simulink model "HoppingRobotModel2"  (R2019b)
settings: Solver=VariableStepAuto  StartTime=0.0  StopTime=10.0  RelTol=1e-3
undefined symbols (not defined in the file): g, I1, I2, ini_theta1, ini_theta1_d, ini_theta2, ini_theta2_d, ini_w, ini_w_d, ini_x0, ini_x0_d, ini_y0, ini_y0_d, M1, M2, r1, r2
settings Model: Creator=fabia  LastModifiedBy=fabia

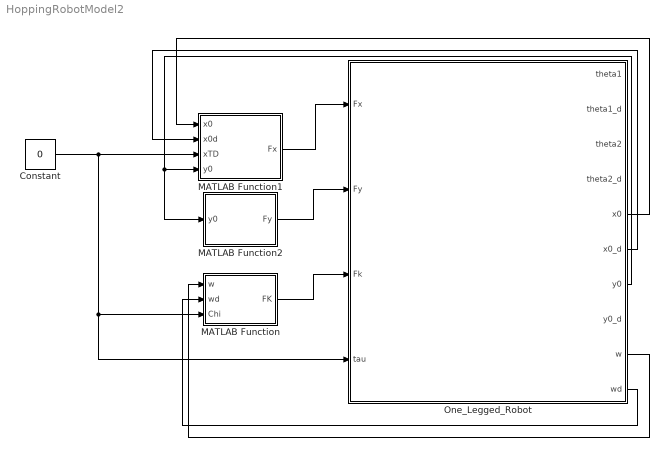
== system HoppingRobotModel2 ==
  Constant : Constant  Value=0
  MATLAB Function : MATLAB Function  TreatAsAtomicUnit=on
  MATLAB Function1 : MATLAB Function  TreatAsAtomicUnit=on
  MATLAB Function2 : MATLAB Function  TreatAsAtomicUnit=on
  One_Legged_Robot : Subsystem
  wires:
  One_Legged_Robot/5(x0) -> MATLAB Function1/1(x0)
  One_Legged_Robot/6(x0_d) -> MATLAB Function1/2(x0d)
  One_Legged_Robot/7(y0) -> MATLAB Function2/1(y0), MATLAB Function1/4(y0)
  One_Legged_Robot/9(w) -> MATLAB Function/1(w)
  One_Legged_Robot/10(wd) -> MATLAB Function/2(wd)
  Constant/1 -> One_Legged_Robot/4(tau), MATLAB Function/3(Chi), MATLAB Function1/3(xTD)
  MATLAB Function1/1(Fx) -> One_Legged_Robot/1(Fx)
  MATLAB Function2/1(Fy) -> One_Legged_Robot/2(Fy)
  MATLAB Function/1(FK) -> One_Legged_Robot/3(Fk)

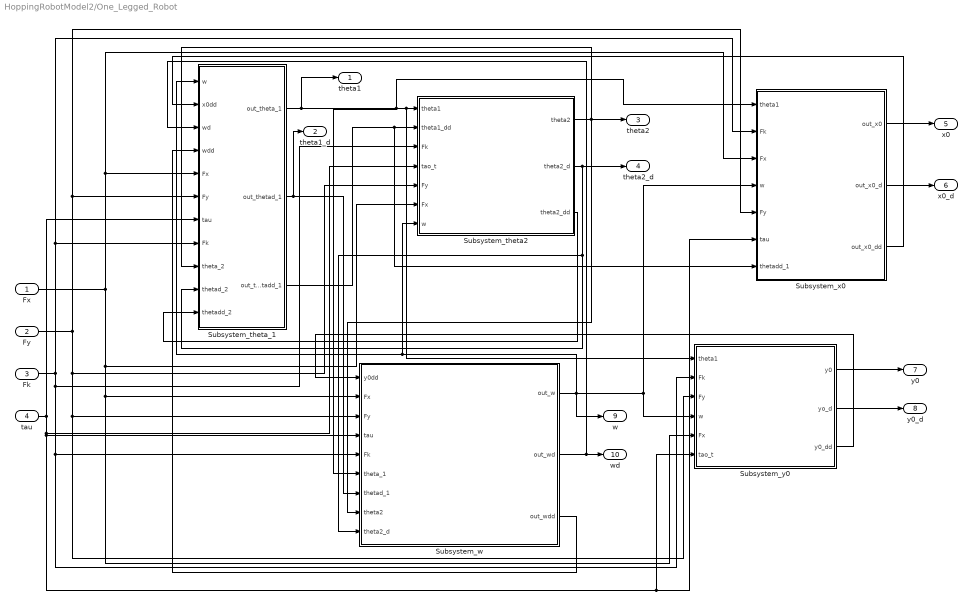
== system HoppingRobotModel2/One_Legged_Robot ==
  Fx : Inport
  Fy : Inport  Port=2
  Fk : Inport  Port=3
  tau : Inport  Port=4
  Subsystem_theta2 : Subsystem
  Subsystem_theta_1 : Subsystem
  Subsystem_w : Subsystem
  Subsystem_x0 : Subsystem
  Subsystem_y0 : Subsystem
  theta1 : Outport
  theta1_d : Outport  Port=2
  theta2 : Outport  Port=3
  theta2_d : Outport  Port=4
  x0 : Outport  Port=5
  x0_d : Outport  Port=6
  y0 : Outport  Port=7
  y0_d : Outport  Port=8
  w : Outport  Port=9
  wd : Outport  Port=10
  wires:
  Subsystem_theta_1/1(out_theta_1) -> theta1/1, Subsystem_y0/1(theta1), Subsystem_theta2/1(theta1), Subsystem_w/6(theta_1), Subsystem_x0/1(theta1)
  Subsystem_theta_1/3(out_thetadd_1) -> Subsystem_x0/7(thetadd_1), Subsystem_theta2/2(theta1_dd)
  Subsystem_theta_1/2(out_thetad_1) -> theta1_d/1, Subsystem_w/7(thetad_1)
  Subsystem_theta2/1(theta2) -> theta2/1, Subsystem_theta_1/9(theta_2), Subsystem_w/8(theta2)
  Subsystem_theta2/2(theta2_d) -> theta2_d/1, Subsystem_theta_1/10(thetad_2), Subsystem_w/9(theta2_d)
  Subsystem_theta2/3(theta2_dd) -> Subsystem_theta_1/11(thetadd_2)
  Subsystem_x0/3(out_x0_dd) -> Subsystem_theta_1/2(x0dd)
  Subsystem_w/1(out_w) -> w/1, Subsystem_x0/4(w), Subsystem_y0/4(w), Subsystem_theta2/7(w), Subsystem_theta_1/1(w)
  Subsystem_w/2(out_wd) -> wd/1, Subsystem_theta_1/3(wd)
  Subsystem_w/3(out_wdd) -> Subsystem_theta_1/4(wdd)
  Subsystem_y0/3(y0_dd) -> Subsystem_w/1(y0dd)
  Fx/1 -> Subsystem_x0/3("Fx "), Subsystem_theta_1/5(Fx), Subsystem_y0/5(Fx), Subsystem_w/2(Fx), Subsystem_theta2/6(Fx)
  Fy/1 -> Subsystem_x0/5("Fy "), Subsystem_theta_1/6(Fy), Subsystem_w/3(Fy), Subsystem_y0/3(Fy), Subsystem_theta2/5(Fy)
  Fk/1 -> Subsystem_w/5(Fk), Subsystem_y0/2(Fk), Subsystem_theta2/3(Fk), Subsystem_theta_1/8(Fk), Subsystem_x0/2(Fk)
  tau/1 -> Subsystem_theta_1/7(tau), Subsystem_y0/6(tao_t), Subsystem_x0/6(tau), Subsystem_w/4(tau), Subsystem_theta2/4(tao_t)
  Subsystem_x0/1("out_x0 ") -> x0/1
  Subsystem_x0/2(out_x0_d) -> x0_d/1
  Subsystem_y0/1(y0) -> y0/1
  Subsystem_y0/2(yo_d) -> y0_d/1

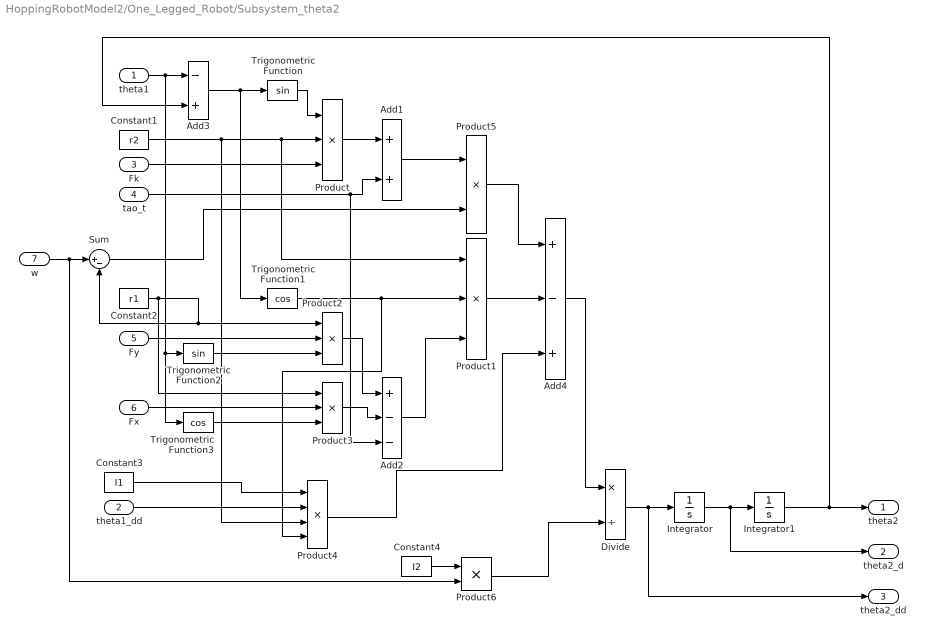
== system HoppingRobotModel2/One_Legged_Robot/Subsystem_theta2 ==
  theta1 : Inport
  theta1_dd : Inport  Port=2
  Fk : Inport  Port=3
  tao_t : Inport  Port=4
  Fy : Inport  Port=5
  Fx : Inport  Port=6
  w : Inport  Port=7
  Add1 : Sum
  Add2 : Sum  Inputs=+--
  Add3 : Sum  Inputs=-+
  Add4 : Sum  Inputs=+-+
  Constant1 : Constant  Value=r2
  Constant2 : Constant  Value=r1
  Constant3 : Constant  Value=I1
  Constant4 : Constant  Value=I2
  Divide : Product  Inputs=*/
  Integrator : Integrator  InitialCondition=ini_theta2_d
  Integrator1 : Integrator  InitialCondition=ini_theta2  LimitOutput=on  UpperSaturationLimit=pi/4  LowerSaturationLimit=-pi/4
  Product{,1..3} (4 alike) : Product  Inputs=3
  Product4 : Product  Inputs=4
  Product5 : Product
  Product6 : Product
  Sum : Sum  Inputs=|+-
  Trigonometric Function : Trigonometry
  Trigonometric Function1 : Trigonometry  Operator=cos
  Trigonometric Function2 : Trigonometry
  Trigonometric Function3 : Trigonometry  Operator=cos
  theta2 : Outport  VectorParamsAs1DForOutWhenUnconnected=off
  theta2_d : Outport  Port=2  VectorParamsAs1DForOutWhenUnconnected=off
  theta2_dd : Outport  Port=3  VectorParamsAs1DForOutWhenUnconnected=off
  wires:
  Fk/1 -> Product/3
  Product1/1 -> Add4/2
  Product2/1 -> Add2/1
  Product5/1 -> Add4/1
  Add4/1 -> Divide/1
  Add3/1 -> Trigonometric Function1/1, Trigonometric Function/1
  Trigonometric Function1/1 -> Product4/4, Product1/2
  Product/1 -> Add1/1
  Constant3/1 -> Product4/1
  Fx/1 -> Product3/2
  Add2/1 -> Product1/3
  Product3/1 -> Add2/2
  Constant1/1 -> Product4/3, Product1/1, Product/2
  Trigonometric Function3/1 -> Product3/3
  Constant2/1 -> Product3/1, Sum/2, Product2/1
  Trigonometric Function2/1 -> Product2/3
  Fy/1 -> Product2/2
  Integrator1/1 -> Add3/2, theta2/1
  Trigonometric Function/1 -> Product/1
  Add1/1 -> Product5/1
  tao_t/1 -> Add2/3, Add1/2
  theta1_dd/1 -> Product4/2
  theta1/1 -> Trigonometric Function3/1, Trigonometric Function2/1, Add3/1
  w/1 -> Product6/2, Sum/1
  Sum/1 -> Product5/2
  Product4/1 -> Add4/3
  Constant4/1 -> Product6/1
  Product6/1 -> Divide/2
  Divide/1 -> theta2_dd/1, Integrator/1
  Integrator/1 -> theta2_d/1, Integrator1/1

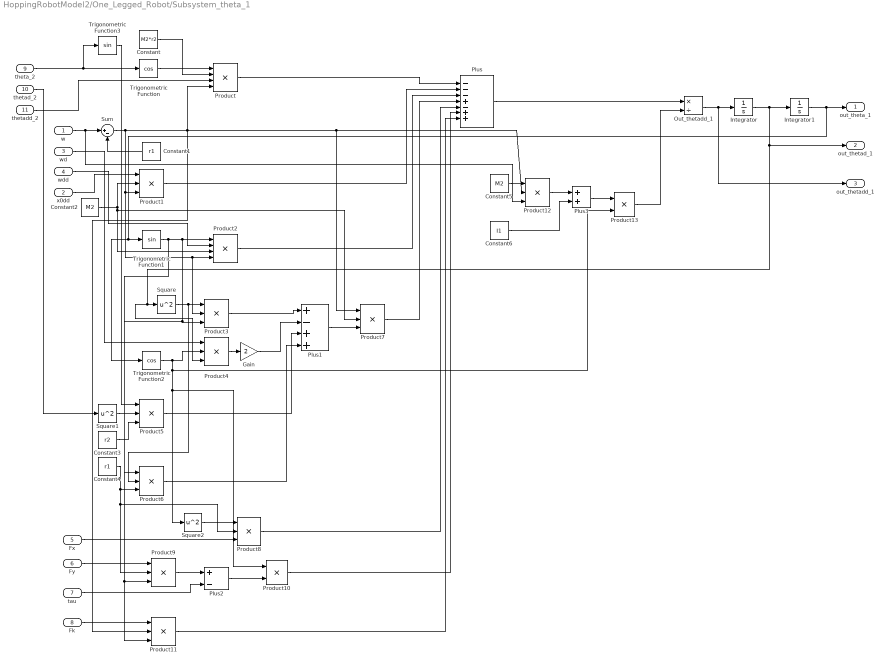
== system HoppingRobotModel2/One_Legged_Robot/Subsystem_theta_1 ==
  w : Inport
  x0dd : Inport  Port=2
  wd : Inport  Port=3
  wdd : Inport  Port=4
  Fx : Inport  Port=5
  Fy : Inport  Port=6
  tau : Inport  Port=7
  Fk : Inport  Port=8
  theta_2 : Inport  Port=9
  thetad_2 : Inport  Port=10
  thetadd_2 : Inport  Port=11
  Constant : Constant  Value=M2*r2
  Constant1 : Constant  Value=r1
  Constant2 : Constant  Value=M2
  Constant3 : Constant  Value=r2
  Constant4 : Constant  Value=r1
  Constant5 : Constant  Value=M2
  Constant6 : Constant  Value=I1
  Gain : Gain  Gain=2
  Integrator : Integrator  InitialCondition=ini_theta1_d
  Integrator1 : Integrator  InitialCondition=ini_theta1  LimitOutput=on  UpperSaturationLimit=pi/4  LowerSaturationLimit=-pi/4
  Out_thetadd_1 : Product  Inputs=*/
  Plus : Sum  Inputs=---+-++
  Plus1 : Sum  Inputs=+-++
  Plus2 : Sum  Inputs=+-
  Plus3 : Sum
  Product : Product  Inputs=4
  Product{1,3..9,11..12} (10 alike) : Product  Inputs=3
  Product10 : Product
  Product13 : Product
  Product2 : Product  Inputs=4
  Square : Math  Operator=square  SignedPower=off  SaturateOnIntegerOverflow=on
  Square1 : Math  Operator=square  SignedPower=off  SaturateOnIntegerOverflow=on
  Square2 : Math  Operator=square  SignedPower=off  SaturateOnIntegerOverflow=on
  Sum : Sum  Inputs=|+-
  Trigonometric Function : Trigonometry  Operator=cos
  Trigonometric Function1 : Trigonometry
  Trigonometric Function2 : Trigonometry  Operator=cos
  Trigonometric Function3 : Trigonometry
  out_theta_1 : Outport
  out_thetad_1 : Outport  Port=2
  out_thetadd_1 : Outport  Port=3
  wires:
  Trigonometric Function/1 -> Product/1
  Constant/1 -> Product/2
  Out_thetadd_1/1 -> out_thetadd_1/1, Integrator/1
  w/1 -> Product12/3, Sum/1
  Sum/1 -> Product2/4, Product3/2, Product1/3, Product11/2, Product12/2, Product7/1, Product/4
  x0dd/1 -> Product1/1
  Constant2/1 -> Product7/2, Product2/3, Product1/2
  Product/1 -> Plus/1
  Product1/1 -> Plus/2
  Trigonometric Function1/1 -> Product9/3, Product11/3, Product6/1, Product3/3, Product2/1
  Integrator1/1 -> Trigonometric Function2/1, Trigonometric Function1/1, out_theta_1/1
  wdd/1 -> Product2/2
  Product2/1 -> Plus/3
  Constant1/1 -> Sum/2
  Square/1 -> Product6/2, Product3/1
  Integrator/1 -> out_thetad_1/1, Product4/3, Square/1, Integrator1/1
  Product3/1 -> Plus1/1
  wd/1 -> Product4/1
  Trigonometric Function2/1 -> Product4/2, Product13/2, Product10/1, Square2/1
  Product4/1 -> Gain/1
  Gain/1 -> Plus1/2
  Trigonometric Function3/1 -> Product5/1
  Square1/1 -> Product5/2
  Constant3/1 -> Product5/3
  Product5/1 -> Plus1/3
  Constant4/1 -> Product9/2, Product8/2, Product6/3
  Product6/1 -> Plus1/4
  Plus1/1 -> Product7/3
  Product7/1 -> Plus/4
  Square2/1 -> Product8/1
  Fx/1 -> Product8/3
  Product8/1 -> Plus/5
  Fy/1 -> Product9/1
  Product9/1 -> Plus2/1
  tau/1 -> Plus2/2
  Plus2/1 -> Product10/2
  Product10/1 -> Plus/6
  Fk/1 -> Product11/1
  Product11/1 -> Plus/7
  Plus/1 -> Out_thetadd_1/1
  Constant5/1 -> Product12/1
  Product12/1 -> Plus3/1
  Constant6/1 -> Plus3/2
  Plus3/1 -> Product13/1
  Product13/1 -> Out_thetadd_1/2
  thetadd_2/1 -> Product/3
  theta_2/1 -> Trigonometric Function3/1, Trigonometric Function/1
  thetad_2/1 -> Square1/1

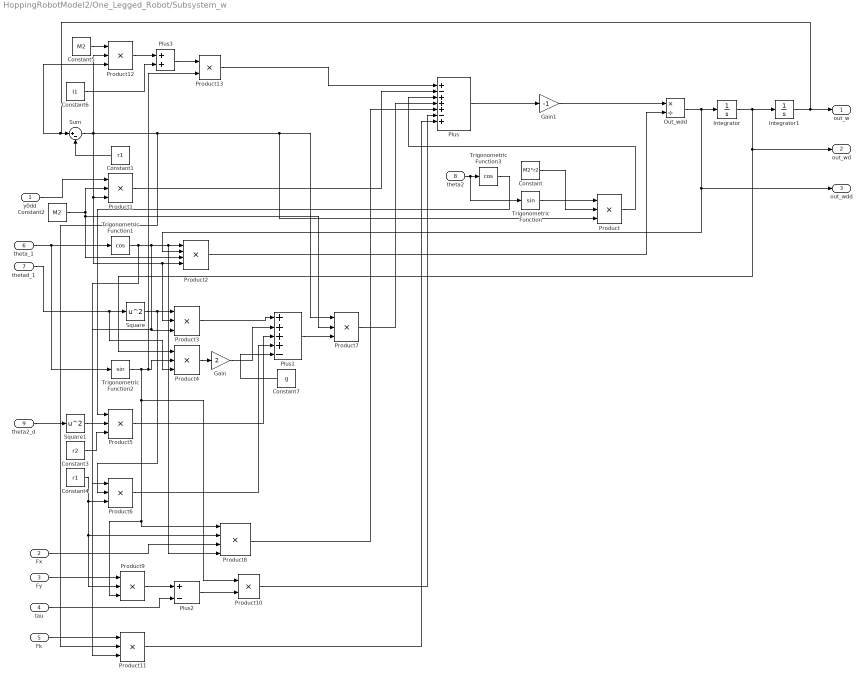
== system HoppingRobotModel2/One_Legged_Robot/Subsystem_w ==
  y0dd : Inport
  Fx : Inport  Port=2
  Fy : Inport  Port=3
  tau : Inport  Port=4
  Fk : Inport  Port=5
  theta_1 : Inport  Port=6
  thetad_1 : Inport  Port=7
  theta2 : Inport  Port=8
  theta2_d : Inport  Port=9
  Constant : Constant  Value=M2*r2
  Constant1 : Constant  Value=r1
  Constant2 : Constant  Value=M2
  Constant3 : Constant  Value=r2
  Constant4 : Constant  Value=r1
  Constant5 : Constant  Value=M2
  Constant6 : Constant  Value=I1
  Constant7 : Constant  Value=g
  Gain : Gain  Gain=2
  Gain1 : Gain  Gain=-1
  Integrator : Integrator  InitialCondition=ini_w_d
  Integrator1 : Integrator  InitialCondition=ini_w  UpperSaturationLimit=pi/4  LowerSaturationLimit=-pi/4
  Out_wdd : Product  Inputs=*/
  Plus : Sum  Inputs=+-+++-+
  Plus1 : Sum  Inputs=++++-
  Plus2 : Sum  Inputs=+-
  Plus3 : Sum
  Product{,1,3..7,9,11..12} (10 alike) : Product  Inputs=3
  Product10 : Product
  Product13 : Product
  Product2 : Product  Inputs=4
  Product8 : Product  Inputs=4
  Square : Math  Operator=square  SignedPower=off  SaturateOnIntegerOverflow=on
  Square1 : Math  Operator=square  SignedPower=off  SaturateOnIntegerOverflow=on
  Sum : Sum  Inputs=|+-
  Trigonometric Function : Trigonometry
  Trigonometric Function1 : Trigonometry  Operator=cos
  Trigonometric Function2 : Trigonometry
  Trigonometric Function3 : Trigonometry  Operator=cos
  out_w : Outport
  out_wd : Outport  Port=2
  out_wdd : Outport  Port=3
  wires:
  Integrator1/1 -> Product12/3, Sum/1, out_w/1
  Sum/1 -> Product12/2, Product2/4, Product3/2, Product1/3, Product11/2, Product/3, Product7/1
  y0dd/1 -> Product1/1
  Constant2/1 -> Product7/2, Product2/3, Product1/2
  Product1/1 -> Plus/2
  Trigonometric Function1/1 -> Product2/1, Product8/4, Product6/1, Product3/3, Product11/3
  Out_wdd/1 -> out_wdd/1, Product2/2, Integrator/1
  Constant1/1 -> Sum/2
  Square/1 -> Product6/2, Product3/1
  Product3/1 -> Plus1/1
  Integrator/1 -> Product4/1, out_wd/1, Integrator1/1
  Product4/1 -> Gain/1
  Gain/1 -> Plus1/2
  Square1/1 -> Product5/2
  Constant3/1 -> Product5/3
  Product5/1 -> Plus1/3
  Constant4/1 -> Product9/2, Product8/2, Product6/3
  Product6/1 -> Plus1/4
  Plus1/1 -> Product7/3
  Product7/1 -> Plus/4
  Trigonometric Function2/1 -> Product13/2, Product4/2, Product9/3, Product8/1, Product10/1
  Fx/1 -> Product8/3
  Product8/1 -> Plus/5
  Fy/1 -> Product9/1
  Product9/1 -> Plus2/1
  tau/1 -> Plus2/2
  Plus2/1 -> Product10/2
  Product10/1 -> Plus/6
  Fk/1 -> Product11/1
  Product11/1 -> Plus/7
  Constant5/1 -> Product12/1
  Product12/1 -> Plus3/1
  Plus3/1 -> Product13/1
  Constant/1 -> Product/2
  Constant6/1 -> Plus3/2
  theta_1/1 -> Trigonometric Function2/1, Trigonometric Function1/1
  thetad_1/1 -> Product4/3, Square/1
  Product13/1 -> Plus/1
  Trigonometric Function/1 -> Product/1
  Trigonometric Function3/1 -> Product5/1
  Constant7/1 -> Plus1/5
  Plus/1 -> Gain1/1
  Gain1/1 -> Out_wdd/1
  theta2/1 -> Trigonometric Function/1, Trigonometric Function3/1
  theta2_d/1 -> Square1/1
  Product/1 -> Plus/3
  Product2/1 -> Out_wdd/2

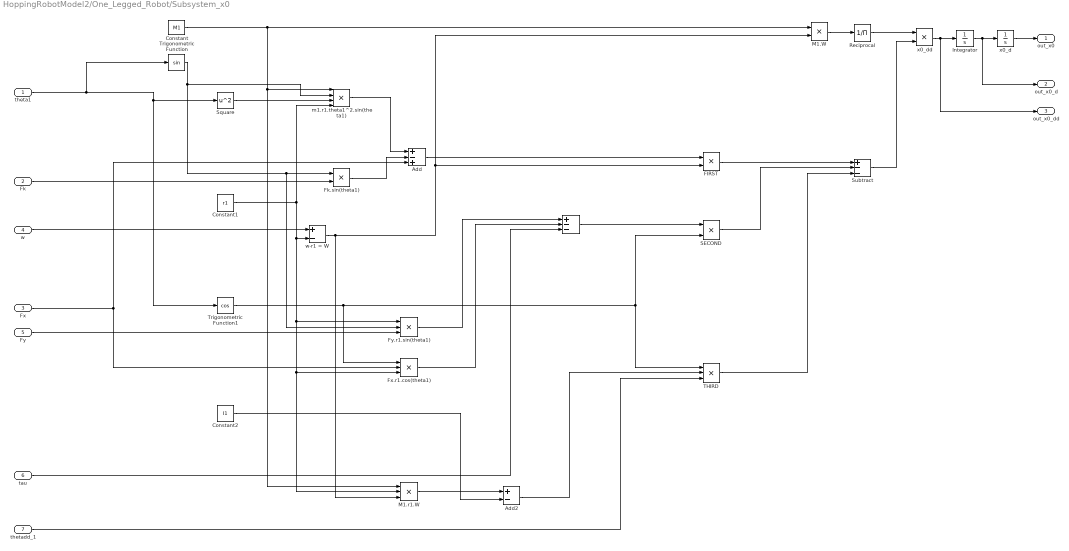
== system HoppingRobotModel2/One_Legged_Robot/Subsystem_x0 ==
  theta1 : Inport
  Fk : Inport  Port=2
  "Fx " : Inport  Port=3
  w : Inport  Port=4
  "Fy " : Inport  Port=5
  tau : Inport  Port=6
  thetadd_1 : Inport  Port=7
  " SECOND" : Product
  " " : Sum  Inputs=+--
  Add : Sum  Inputs=+-+
  Add2 : Sum  Inputs=+-
  Constant : Constant  Value=M1
  Constant1 : Constant  Value=r1
  Constant2 : Constant  Value=I1
  FIRST : Product
  Fk.sin(theta1) : Product
  Fx.r1.cos(theta1) : Product  Inputs=3
  Fy.r1.sin(theta1) : Product  Inputs=3
  Integrator : Integrator  InitialCondition=ini_x0_d
  M1.W : Product
  M1.r1.W : Product  Inputs=3
  Reciprocal : Product  Inputs=/
  Square : Math  Operator=square  SignedPower=off  SaturateOnIntegerOverflow=on
  Subtract : Sum  Inputs=+--
  "THIRD " : Product  Inputs=3
  Trigonometric Function : Trigonometry
  Trigonometric Function1 : Trigonometry  Operator=cos
  m1.r1.theta1^2.sin(theta1) : Product  Inputs=4
  w-r1 = W : Sum  Inputs=+-
  x0_d : Integrator  InitialCondition=ini_x0
  "x0_dd " : Product
  "out_x0 " : Outport
  out_x0_d : Outport  Port=2
  out_x0_dd : Outport  Port=3
  wires:
  Add/1 -> FIRST/1
  Constant1/1 -> m1.r1.theta1^2.sin(theta1)/4, M1.r1.W/2, Fx.r1.cos(theta1)/3, Fy.r1.sin(theta1)/1, w-r1 = W/2
  w/1 -> w-r1 = W/1
  Reciprocal/1 -> "x0_dd "/1
  thetadd_1/1 -> "THIRD "/3
  Trigonometric Function1/1 -> "THIRD "/1, " SECOND"/2, Fx.r1.cos(theta1)/1
  m1.r1.theta1^2.sin(theta1)/1 -> Add/1
  tau/1 -> " "/3
  M1.r1.W/1 -> Add2/1
  Square/1 -> m1.r1.theta1^2.sin(theta1)/3
  Trigonometric Function/1 -> Fy.r1.sin(theta1)/2, Fk.sin(theta1)/1, m1.r1.theta1^2.sin(theta1)/2
  Constant/1 -> m1.r1.theta1^2.sin(theta1)/1, M1.r1.W/1, M1.W/1
  Constant2/1 -> Add2/2
  FIRST/1 -> Subtract/1
  theta1/1 -> Trigonometric Function1/1, Square/1, Trigonometric Function/1
  "x0_dd "/1 -> out_x0_dd/1, Integrator/1
  "Fx "/1 -> Fx.r1.cos(theta1)/2, Add/3
  Fx.r1.cos(theta1)/1 -> " "/2
  x0_d/1 -> "out_x0 "/1
  w-r1 = W/1 -> FIRST/2, M1.W/2, M1.r1.W/3
  Add2/1 -> "THIRD "/2
  Integrator/1 -> out_x0_d/1, x0_d/1
  Fy.r1.sin(theta1)/1 -> " "/1
  "Fy "/1 -> Fy.r1.sin(theta1)/3
  M1.W/1 -> Reciprocal/1
  "THIRD "/1 -> Subtract/3
  " SECOND"/1 -> Subtract/2
  Fk/1 -> Fk.sin(theta1)/2
  Fk.sin(theta1)/1 -> Add/2
  " "/1 -> " SECOND"/1
  Subtract/1 -> "x0_dd "/2

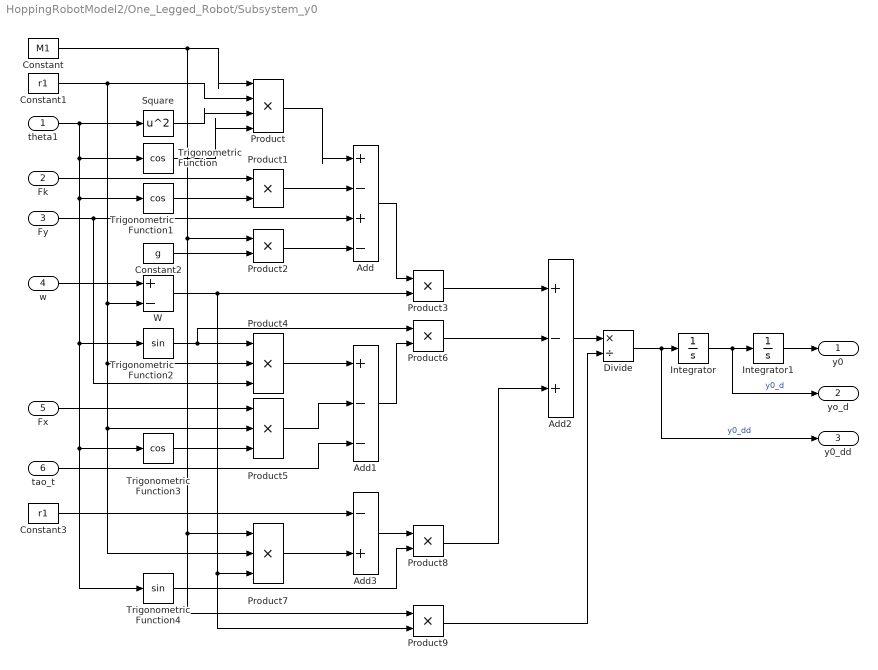
== system HoppingRobotModel2/One_Legged_Robot/Subsystem_y0 ==
  theta1 : Inport
  Fk : Inport  Port=2
  Fy : Inport  Port=3
  w : Inport  Port=4
  Fx : Inport  Port=5
  tao_t : Inport  Port=6
  Add : Sum  Inputs=+-+-
  Add1 : Sum  Inputs=+--
  Add2 : Sum  Inputs=+-+
  Add3 : Sum  Inputs=-+
  Constant : Constant  Value=M1
  Constant1 : Constant  Value=r1
  Constant2 : Constant  Value=g
  Constant3 : Constant  Value=r1
  Divide : Product  Inputs=*/
  Integrator : Integrator  InitialCondition=ini_y0_d
  Integrator1 : Integrator  InitialCondition=ini_y0
  Product : Product  Inputs=4
  Product{1..3,6,8..9} (6 alike) : Product
  Product4 : Product  Inputs=3
  Product5 : Product  Inputs=3
  Product7 : Product  Inputs=3
  Square : Math  Operator=square  SaturateOnIntegerOverflow=on
  Trigonometric Function : Trigonometry  Operator=cos
  Trigonometric Function1 : Trigonometry  Operator=cos
  Trigonometric Function2 : Trigonometry
  Trigonometric Function3 : Trigonometry  Operator=cos
  Trigonometric Function4 : Trigonometry
  W : Sum  Inputs=+-
  y0 : Outport  VectorParamsAs1DForOutWhenUnconnected=off
  yo_d : Outport  Port=2  VectorParamsAs1DForOutWhenUnconnected=off
  y0_dd : Outport  Port=3  VectorParamsAs1DForOutWhenUnconnected=off
  wires:
  Integrator/1 -> yo_d/1, Integrator1/1  "y0_d"
  Add2/1 -> Divide/1
  Square/1 -> Product/3
  Integrator1/1 -> y0/1
  Divide/1 -> y0_dd/1, Integrator/1  "y0_dd"
  Product8/1 -> Add2/3
  Product6/1 -> Add2/2
  Add3/1 -> Product8/1
  Trigonometric Function4/1 -> Product8/2
  Product7/1 -> Add3/2
  Product9/1 -> Divide/2
  Add1/1 -> Product6/2
  W/1 -> Product7/3, Product9/2, Product3/2
  Constant2/1 -> Product2/2
  Trigonometric Function1/1 -> Product1/2
  Product/1 -> Add/1
  Fy/1 -> Product4/3, Add/3
  w/1 -> W/1
  Add/1 -> Product3/1
  Fk/1 -> Product1/1
  Product4/1 -> Add1/1
  Fx/1 -> Product5/1
  Product1/1 -> Add/2
  Constant/1 -> Product9/1, Product7/1, Product2/1, Product/1
  Trigonometric Function/1 -> Product/4
  Trigonometric Function3/1 -> Product5/3
  Constant1/1 -> Product7/2, Product5/2, Product4/2, W/2, Product/2
  Product2/1 -> Add/4
  tao_t/1 -> Add1/3
  Trigonometric Function2/1 -> Product6/1, Product4/1
  Product5/1 -> Add1/2
  Constant3/1 -> Add3/1
  theta1/1 -> Trigonometric Function4/1, Trigonometric Function3/1, Trigonometric Function2/1, Trigonometric Function1/1, Trigonometric Function/1, Square/1
  Product3/1 -> Add2/1

== matlab function HoppingRobotModel2/MATLAB Function1 ==
  data: x0 input; Fx output; x0d input; xTD input; y0 input
function Fx = fcn(x0,x0d,xTD,y0)
KG=10^4; % [Nt/m]
BG=75; % [Nt-s/m]
if y0<0
   Fx = -KG*(x0-xTD)-(BG*x0d);
else
   Fx=0;
end

== matlab function HoppingRobotModel2/MATLAB Function ==
  data: w input; FK output; wd input; Chi input
function FK = fcn(w,wd,Chi)
k0=1; % [m]
KL=10^3; % [Nt/m]

KL2=10^5; % [Nt/m]
BL2=125; % [Nt-s/m]
if (k0-w+Chi)>0
   FK = KL*(k0-w+Chi);
else
    FK=KL2*(k0-w+Chi)-(BL2*wd);
end

== matlab function HoppingRobotModel2/MATLAB Function2 ==
  data: Fy output; y0 input
function Fy = fcn(y0)
KG=10^4; % [Nt/m]
BG=75; % [Nt-s/m]
if y0<0
   Fy = (-KG*y0)-(BG*y0);
else
    Fy=0;
end
